simulink model "compensatore_dinamico_sinusoide"  (R2018a)
settings: Solver=VariableStepAuto  StartTime=0.0  StopTime=50  RelTol=1e-3
undefined symbols (not defined in the file): A, alpha_eq, AO, B, BO, CO, dati, DO, fd, fd_eq, input, K, x0, x_eq
settings Model: Creator=Ivonne  LastModifiedBy=Ivonne

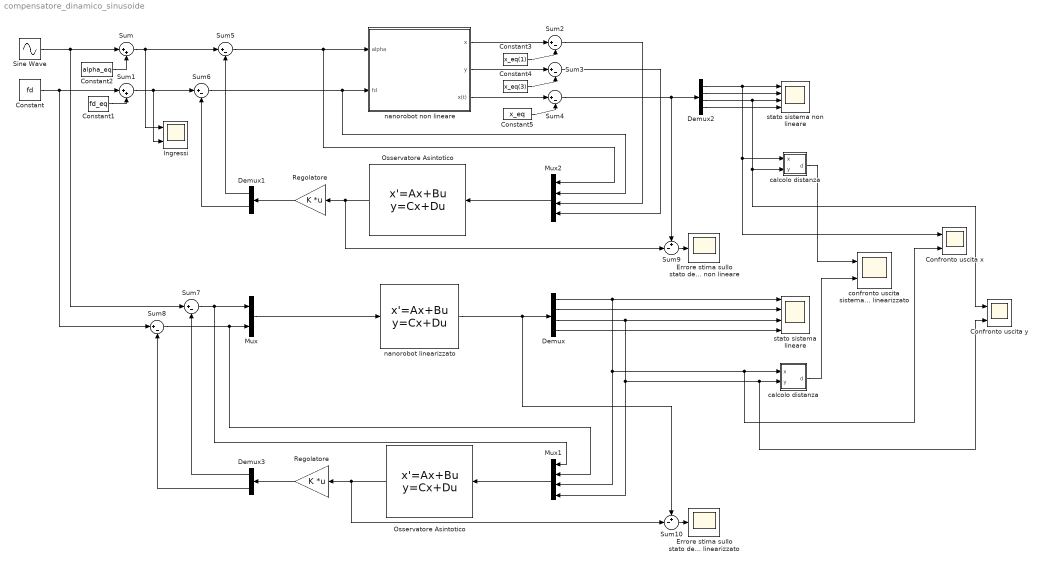
== system compensatore_dinamico_sinusoide ==
  Confronto uscita x : Scope  NumInputPorts=2
  Confronto uscita y : Scope  NumInputPorts=2
  Constant : Constant  Value=fd
  Constant1 : Constant  Value=fd_eq
  Constant2 : Constant  Value=alpha_eq
  Constant3 : Constant  Value=x_eq(1)
  Constant4 : Constant  Value=x_eq(3)
  Constant5 : Constant  Value=x_eq
  Demux : Demux
  Demux1 : Demux  Outputs=2
  Demux2 : Demux
  Demux3 : Demux  Outputs=2
  Errore stima sullo stato del modello linearizzato : Scope
  Errore stima sullo stato del modello non lineare : Scope
  Ingressi : Scope  NumInputPorts=2
  Mux : Mux  Inputs=2
  Mux1 : Mux
  Mux2 : Mux
  Osservatore Asintotico : StateSpace  A=AO  B=BO  C=CO  D=DO  InitialCondition=input
  "Osservatore Asintotico " : StateSpace  A=AO  B=BO  C=CO  D=DO  InitialCondition=input
  "Regolatore " : Gain  Gain=K  Multiplication=Matrix(K*u)
  "Regolatore " : Gain  Gain=K  Multiplication=Matrix(K*u)
  Sine Wave : Sin  SampleTime=0
  Sum : Sum  Inputs=|++
  Sum1 : Sum  Inputs=|++
  Sum10 : Sum  Inputs=+-|
  Sum{2..8} (7 alike) : Sum  Inputs=|+-
  Sum9 : Sum  Inputs=+-|
  "calcolo distanza " : Subsystem
  "calcolo distanza " : Subsystem
  confronto uscita sistema non lineare e modello linearizzato : Scope  NumInputPorts=2
  nanorobot linearizzato : StateSpace  A=A  B=B  C=eye(4)  D=zeros(4,2)  InitialCondition=x0
  nanorobot non lineare : Subsystem
  stato sistema lineare : Scope  NumInputPorts=4
  stato sistema non lineare : Scope  NumInputPorts=4
  wires:
  Constant2/1 -> Sum/2
  Constant1/1 -> Sum1/2
  Mux/1 -> nanorobot linearizzato/1
  nanorobot linearizzato/1 -> Demux/1, Sum10/1
  Constant3/1 -> Sum2/2
  nanorobot non lineare/1(x) -> Sum2/1
  Sum2/1 -> Mux2/3
  nanorobot non lineare/2(y) -> Sum3/1
  Constant4/1 -> Sum3/2
  Sum3/1 -> Mux2/4
  Sine Wave/1 -> Sum/1, Sum7/1
  nanorobot non lineare/3(x(t)) -> Sum4/1
  Constant5/1 -> Sum4/2
  Demux2/4 -> stato sistema non lineare/4
  Demux2/1 -> stato sistema non lineare/1, Confronto uscita x/1, "calcolo distanza "/1(x)
  Demux2/2 -> stato sistema non lineare/2
  Demux2/3 -> stato sistema non lineare/3, Confronto uscita y/1, "calcolo distanza "/2(y)
  Sum/1 -> Ingressi/1, Sum5/1
  Sum1/1 -> Ingressi/2, Sum6/1
  Sum5/1 -> Mux2/1, nanorobot non lineare/1(alpha)
  Sum6/1 -> Mux2/2, nanorobot non lineare/2(fd)
  "Regolatore "/1 -> Demux1/1
  Demux1/1 -> Sum5/2
  Demux1/2 -> Sum6/2
  Sum7/1 -> Mux/1, Mux1/1
  Sum8/1 -> Mux1/2, Mux/2
  "Regolatore "/1 -> Demux3/1
  Demux3/1 -> Sum7/2
  Demux3/2 -> Sum8/2
  Demux/1 -> Mux1/3, Confronto uscita x/2, "calcolo distanza "/1(x), stato sistema lineare/1
  Demux/3 -> Mux1/4, Confronto uscita y/2, "calcolo distanza "/2(y), stato sistema lineare/3
  Demux/2 -> stato sistema lineare/2
  Demux/4 -> stato sistema lineare/4
  Sum4/1 -> Demux2/1, Sum9/1
  Constant/1 -> Sum8/1, Sum1/1
  Osservatore Asintotico/1 -> Sum10/2, "Regolatore "/1
  Mux1/1 -> Osservatore Asintotico/1
  Mux2/1 -> "Osservatore Asintotico "/1
  "Osservatore Asintotico "/1 -> Sum9/2, "Regolatore "/1
  Sum9/1 -> Errore stima sullo stato del modello non lineare/1
  Sum10/1 -> Errore stima sullo stato del modello linearizzato/1
  "calcolo distanza "/1(d) -> confronto uscita sistema non lineare e modello linearizzato/1
  "calcolo distanza "/1(d) -> confronto uscita sistema non lineare e modello linearizzato/2

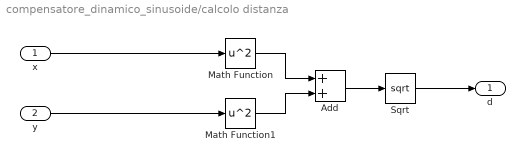
== system compensatore_dinamico_sinusoide/calcolo distanza  ==
  x : Inport
  y : Inport  Port=2
  Add : Sum
  Math Function : Math  Operator=square  SaturateOnIntegerOverflow=on
  Math Function1 : Math  Operator=square  SaturateOnIntegerOverflow=on
  Sqrt : Sqrt  SaturateOnIntegerOverflow=on
  d : Outport
  wires:
  Add/1 -> Sqrt/1
  x/1 -> Math Function/1
  Math Function/1 -> Add/1
  Math Function1/1 -> Add/2
  Sqrt/1 -> d/1
  y/1 -> Math Function1/1

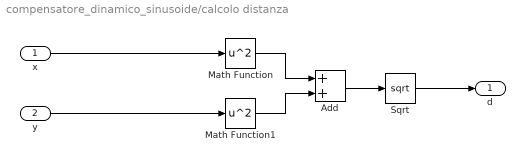
== system compensatore_dinamico_sinusoide/calcolo distanza  ==
  x : Inport
  y : Inport  Port=2
  Add : Sum
  Math Function : Math  Operator=square  SaturateOnIntegerOverflow=on
  Math Function1 : Math  Operator=square  SaturateOnIntegerOverflow=on
  Sqrt : Sqrt  SaturateOnIntegerOverflow=on
  d : Outport
  wires:
  Add/1 -> Sqrt/1
  x/1 -> Math Function/1
  Math Function/1 -> Add/1
  Math Function1/1 -> Add/2
  Sqrt/1 -> d/1
  y/1 -> Math Function1/1

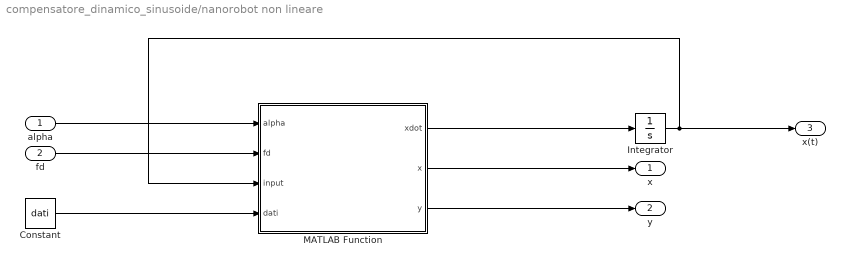
== system compensatore_dinamico_sinusoide/nanorobot non lineare ==
  alpha : Inport
  fd : Inport  Port=2
  Constant : Constant  Value=dati
  Integrator : Integrator  InitialCondition=x0
  MATLAB Function : MATLAB Function  TreatAsAtomicUnit=on
  x : Outport
  y : Outport  Port=2
  x(t) : Outport  Port=3
  wires:
  MATLAB Function/1(xdot) -> Integrator/1
  Integrator/1 -> x(t)/1, MATLAB Function/3(input)
  MATLAB Function/2(x) -> x/1
  Constant/1 -> MATLAB Function/4(dati)
  alpha/1 -> MATLAB Function/1(alpha)
  MATLAB Function/3(y) -> y/1
  fd/1 -> MATLAB Function/2(fd)

== matlab function compensatore_dinamico_sinusoide/nanorobot non lineare/MATLAB Function ==
  data: xdot output; alpha input; fd input; input input; x output; dati input; y output
function [ xdot, x, y ] = fcn(alpha, fd, input, dati)
% input : condizioni iniziali
% u : ingresso del sistema -> [ alpha, fd]
% dati : parametri del modello fisico -> [ R, Fm, m, eta,l, dP, r, vf ]
R= dati(1);                 
Fm = dati(2);  
m = dati(3);
eta = dati(4);
l = dati(5);
dP = dati(6);
r = dati(7);
vf = dati(8);
% variabili di stato 
% x1 = x, x2 = xp -> x1p, x3 = y, x4 = yp -> x3p
% allora xpp = x2p e ypp = x4p
x1 = input(1); % xdot(1) = x2 -> 1/s 
x2 = input(2); % xdot(2) = x2p -> 1/s 
x3 = input(3); % xdot(3) = x4 -> 1/s
x4 = input(4); % xdot(4) = x4p -> 1/s
% forma di stato
xdot = [ x2;
         ((-6*pi*eta*R)/m)*x2 + ((6*pi*eta*R)/m)*vf + (Fm/m)*cos(alpha) + fd/m;
         x4;
         ((-6*pi*eta*R)/m)*x4 + (Fm/m)*sin(alpha)];

% coordinate cartesiane
x = x1;
y = x3;
